simulink model "controlador_pid_discreto"  (R2023b)
settings: Solver=VariableStepAuto  StartTime=0.0  StopTime=10.0  RelTol=1e-3
values from neighbouring files (symbols this model uses):
  ba_num = Jeq_ctrl*n_pid*wn_pid    (= 0.0395694444444)    [controlador_foc_simulink.m]    (also in sistema_completo_en_codigo.m)
  Ksa_num = Jeq_ctrl*n_pid*wn_pid^2    (= 31.6555555556)    [controlador_foc_simulink.m]    (also in sistema_completo_en_codigo.m)
  Ksia_num = Jeq_ctrl*wn_pid^3    (= 10129.7777778)    [controlador_foc_simulink.m]    (also in sistema_completo_en_codigo.m)
undefined symbols (not defined in the file or in its folder): DiscIntNeverNeededParam
settings Model: Creator=Pc  LastModifiedBy=Pc

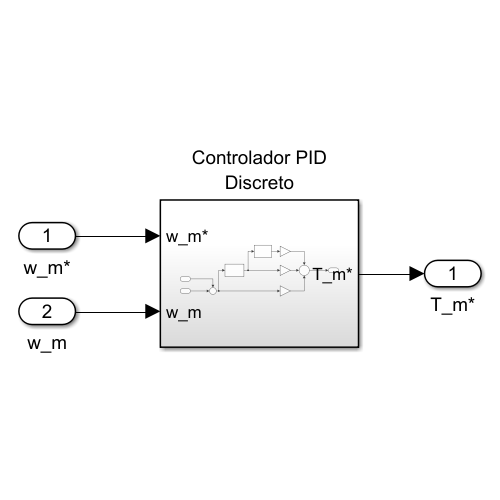
[thumbnail: Simulink's stored preview of the top-level diagram]
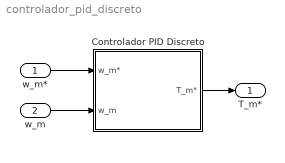
== system controlador_pid_discreto ==
  w_m* : Inport
  w_m : Inport  Port=2
  Controlador PID Discreto : Subsystem
  T_m* : Outport
  wires:
  w_m*/1 -> Controlador PID Discreto/1(w_m*)
  w_m/1 -> Controlador PID Discreto/2(w_m)
  Controlador PID Discreto/1(T_m*) -> T_m*/1

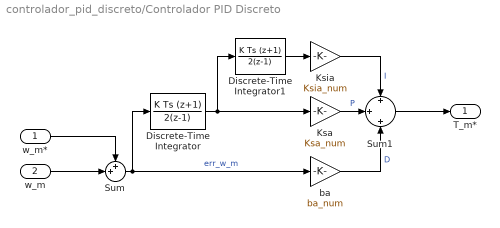
== system controlador_pid_discreto/Controlador PID Discreto ==
  w_m* : Inport
  w_m : Inport  Port=2
  Discrete-Time Integrator : DiscreteIntegrator  IntegratorMethod=Integration: Trapezoidal  SampleTime=-1  ICPrevOutput=DiscIntNeverNeededParam  ICPrevScaledInput=DiscIntNeverNeededParam
  Discrete-Time Integrator1 : DiscreteIntegrator  IntegratorMethod=Integration: Trapezoidal  SampleTime=-1  ICPrevOutput=DiscIntNeverNeededParam  ICPrevScaledInput=DiscIntNeverNeededParam
  Ksa : Gain  Gain=Ksa_num
  Ksia : Gain  Gain=Ksia_num
  Sum : Sum  Inputs=++|
  Sum1 : Sum  Inputs=+|+|+
  ba : Gain  Gain=ba_num
  T_m* : Outport
  wires:
  Sum1/1 -> T_m*/1
  ba/1 -> Sum1/3  "D"
  Sum/1 -> ba/1, Discrete-Time Integrator/1  "err_w_m"
  Discrete-Time Integrator1/1 -> Ksia/1
  w_m*/1 -> Sum/1
  Discrete-Time Integrator/1 -> Ksa/1, Discrete-Time Integrator1/1
  w_m/1 -> Sum/2
  Ksia/1 -> Sum1/1  "I"
  Ksa/1 -> Sum1/2  "P"
